simulink model "mcb_pmsm_foc_sim_RL"  (R2023a)
settings: Solver=VariableStepAuto  StartTime=0.0  StopTime=2  RelTol=1e-3
undefined symbols (not defined in the file): dataType, DiscIntNeverNeededParam, inverter, PI_params, pmsm, PU_System, Ts, Ts_agent, Ts_motor, Ts_simulink, Ts_speed
libraries: mcbcontrolslib x8, mcbpositiondecoderlib x3, simulink x2, rllib x1, mcbplantlib x1, autolibpmsmexterior x1, slpidlib x1
settings Model: Creator=The MathWorks, Inc.  LastModifiedBy=awear
settings SolverCC: AlgebraicLoopSolver=TrustRegion
settings OptimizationCC: ReuseModelBlockBuffer=off
settings DebuggingCC: ParameterPrecisionLossMsg=none  UnconnectedInputMsg=warning  UnconnectedOutputMsg=warning  UnconnectedLineMsg=warning
settings ModelReferenceCC: EnableRefExpFcnMdlSchedulingChecks=on
settings RTWCC: DLArmComputeVersion=19.05

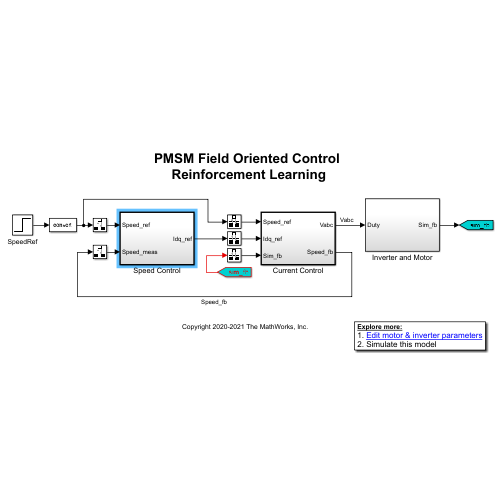
[thumbnail: Simulink's stored preview of the top-level diagram]
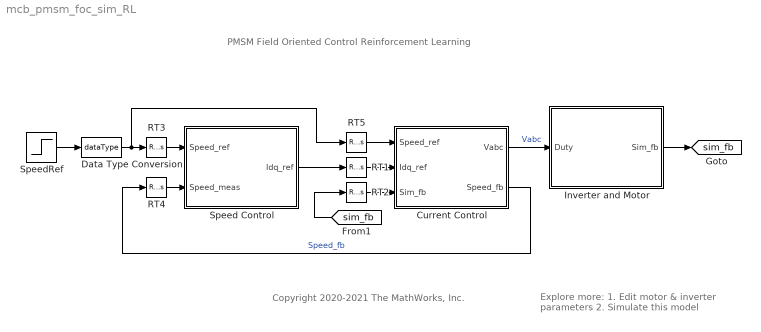
== system mcb_pmsm_foc_sim_RL ==
  note: PMSM Field Oriented Control
      | Reinforcement Learning
  note: Copyright 2020-2021 The MathWorks, Inc.
  note: Explore more:
      | 1. Edit motor & inverter parameters
      | 2. Simulate this model
  Current Control : Subsystem  TreatAsAtomicUnit=on
  Data Type Conversion : DataTypeConversion  OutDataTypeStr=dataType  SaturateOnIntegerOverflow=off  RndMeth=Floor
  Inverter and Motor : Subsystem
  RT1 : RateTransition  Deterministic=off  OutPortSampleTime=Ts
  RT2 : RateTransition  Deterministic=off  OutPortSampleTime=Ts
  RT3 : RateTransition  Deterministic=off  OutPortSampleTime=Ts_speed
  RT4 : RateTransition  Deterministic=off  OutPortSampleTime=Ts_speed
  RT5 : RateTransition  Deterministic=off  OutPortSampleTime=Ts
  Speed Control : Subsystem  TreatAsAtomicUnit=on  SystemSampleTime=Ts_speed
  SpeedRef : Step  Before=0.2  After=0.6  OutDataTypeStr=single  SampleTime=Ts_speed
  tag scope: sim_fb=global
  wires:
  Speed Control/1(Idq_ref) -> RT1/1
  RT5/1 -> Current Control/1(Speed_ref)
  SpeedRef/1 -> Data Type Conversion/1
  Current Control/2(Speed_fb) -> RT4/1  "Speed_fb"
  RT1/1 -> Current Control/2(Idq_ref)
  [sim_fb] -> RT2/1
  Data Type Conversion/1 -> RT5/1, RT3/1
  RT4/1 -> Speed Control/2(Speed_meas)
  Current Control/1(Vabc) -> Inverter and Motor/1(Duty)  "Vabc"
  RT3/1 -> Speed Control/1(Speed_ref)
  Inverter and Motor/1(Sim_fb) -> [sim_fb]
  RT2/1 -> Current Control/3(Sim_fb)

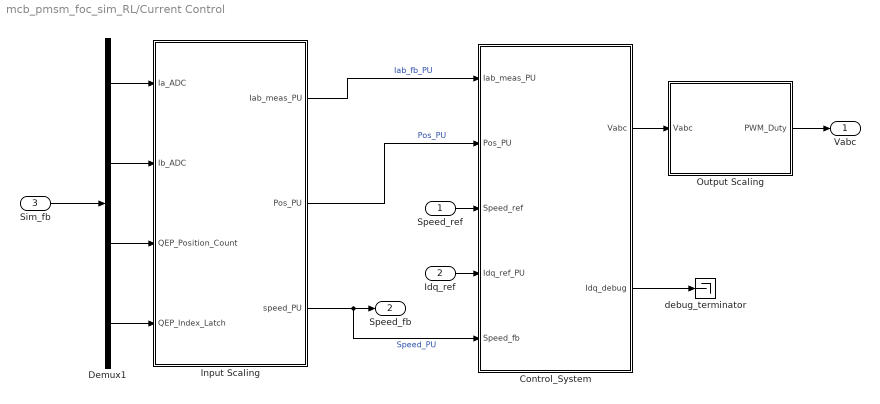
== system mcb_pmsm_foc_sim_RL/Current Control ==
  Speed_ref : Inport
  Idq_ref : Inport  Port=2
  Sim_fb : Inport  Port=3
  Control_System : Subsystem
  Demux1 : Demux
  Input Scaling : Subsystem
  Output Scaling : Subsystem
  debug_terminator : Terminator
  Vabc : Outport  InitialOutput=0  VectorParamsAs1DForOutWhenUnconnected=off
  Speed_fb : Outport  Port=2  InitialOutput=0  VectorParamsAs1DForOutWhenUnconnected=off
  wires:
  Input Scaling/2(Pos_PU) -> Control_System/2(Pos_PU)  "Pos_PU"
  Input Scaling/3(speed_PU) -> Control_System/5(Speed_fb), Speed_fb/1  "Speed_PU"
  Demux1/1 -> Input Scaling/1(Ia_ADC)
  Demux1/2 -> Input Scaling/2(Ib_ADC)
  Demux1/3 -> Input Scaling/3(QEP_Position_Count)
  Demux1/4 -> Input Scaling/4(QEP_Index_Latch)
  Control_System/2(Idq_debug) -> debug_terminator/1
  Sim_fb/1 -> Demux1/1
  Idq_ref/1 -> Control_System/4(Idq_ref_PU)
  Control_System/1(Vabc) -> Output Scaling/1(Vabc)
  Output Scaling/1(PWM_Duty) -> Vabc/1
  Input Scaling/1(Iab_meas_PU) -> Control_System/1(Iab_meas_PU)  "Iab_fb_PU"
  Speed_ref/1 -> Control_System/3(Speed_ref)

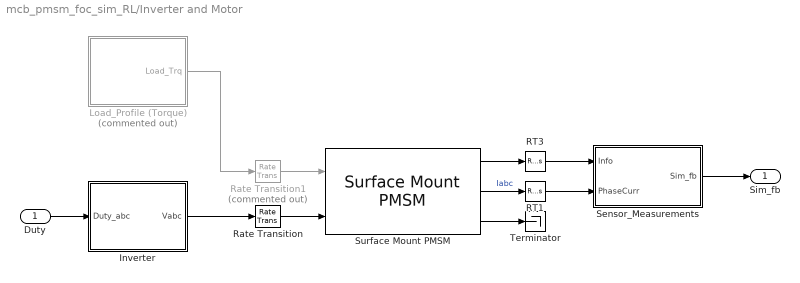
== system mcb_pmsm_foc_sim_RL/Inverter and Motor ==
  Duty : Inport
  Inverter : Subsystem
  Load_Profile (Torque) : Subsystem  Commented=on
  RT1 : RateTransition  Deterministic=off  OutPortSampleTime=Ts_simulink
  RT3 : RateTransition  Deterministic=off  OutPortSampleTime=Ts_simulink
  Rate Transition : RateTransition  Deterministic=off  OutPortSampleTime=Ts_motor
  Rate Transition1 : RateTransition  Commented=on  Deterministic=off  OutPortSampleTime=Ts_motor
  Sensor_Measurements : Subsystem
  Surface Mount PMSM : autolibpmsmexterior/Surface Mount PMSM  port_config=Torque  sim_type=Discrete  Ts=Ts_motor  P=pmsm.p  Rs=pmsm.Rs  Ldq_=pmsm.Ld  KConstText=Permanent flux linkage constant (lambda_pm):  lambda_pm=pmsm.FluxPM  Ke=159.9771  Kt=1.323  mechanical=[pmsm.J, pmsm.B, 0]  idq0=[0 0]  theta_init=0  omega_init=0  KConst=pmsm.FluxPM  lambda_pm_calc=pmsm.FluxPM  RefBlkName='autolibpmsmexterior/Surface Mount PMSM'  aMode=5  Ldq="[0.0002      0.0002]"
  Terminator : Terminator
  Sim_fb : Outport  VectorParamsAs1DForOutWhenUnconnected=off
  wires:
  Surface Mount PMSM/1 -> RT3/1
  RT1/1 -> Sensor_Measurements/2(PhaseCurr)
  RT3/1 -> Sensor_Measurements/1(Info)
  Inverter/1(Vabc) -> Rate Transition/1
  Rate Transition/1 -> Surface Mount PMSM/2
  Surface Mount PMSM/3 -> Terminator/1
  Rate Transition1/1 -> Surface Mount PMSM/1
  Sensor_Measurements/1(Sim_fb) -> Sim_fb/1
  Surface Mount PMSM/2 -> RT1/1  "Iabc"
  Load_Profile (Torque)/1(Load_Trq) -> Rate Transition1/1
  Duty/1 -> Inverter/1(Duty_abc)

== system mcb_pmsm_foc_sim_RL/Speed Control ==
  Speed_ref : Inport
  Speed_meas : Inport  Port=2
  Id_ref : Constant  Value=0  OutDataTypeStr=dataType  SampleTime=Ts_speed
  Mux1 : Mux  Inputs=2
  PI_Controller_Speed : Subsystem
  Speed Tracking : Scope  NumInputPorts=2
  Zero_Cancellation : mcbcontrolslib/IIR Filter  VariantControl=Low Pass Filter  VariantSelect=Low-pass  Filter_constant=0.01*(Ts_speed/Ts)  advancedSettings=off  Ts=50e-6  cutOff_freq=1
  Idq_ref : Outport  VectorParamsAs1DForOutWhenUnconnected=off
  wires:
  Speed_meas/1 -> Speed Tracking/2, PI_Controller_Speed/2(N_fb)  "Speed_fb"
  Id_ref/1 -> Mux1/1
  PI_Controller_Speed/1(Iq_ref) -> Mux1/2
  Mux1/1 -> Idq_ref/1
  Zero_Cancellation/1 -> PI_Controller_Speed/1(N_ref)
  Speed_ref/1 -> Speed Tracking/1, Zero_Cancellation/1  "Speed_Ref"

== system mcb_pmsm_foc_sim_RL/Current Control/Control_System ==
  Iab_meas_PU : Inport
  Pos_PU : Inport  Port=2
  Speed_ref : Inport  Port=3
  Idq_ref_PU : Inport  Port=4
  Speed_fb : Inport  Port=5
  Closed Loop Control : Subsystem
  Vabc : Outport  VectorParamsAs1DForOutWhenUnconnected=off
  Idq_debug : Outport  Port=2  VectorParamsAs1DForOutWhenUnconnected=off
  wires:
  Iab_meas_PU/1 -> Closed Loop Control/1(Iab_meas_PU)
  Pos_PU/1 -> Closed Loop Control/2(Pos_PU)
  Idq_ref_PU/1 -> Closed Loop Control/3(Idq_ref_PU)
  Closed Loop Control/1(Idq_debug) -> Idq_debug/1
  Closed Loop Control/2(Vabc in PU) -> Vabc/1
  Speed_ref/1 -> Closed Loop Control/4(Speed_ref)
  Speed_fb/1 -> Closed Loop Control/5(Speef_fb)

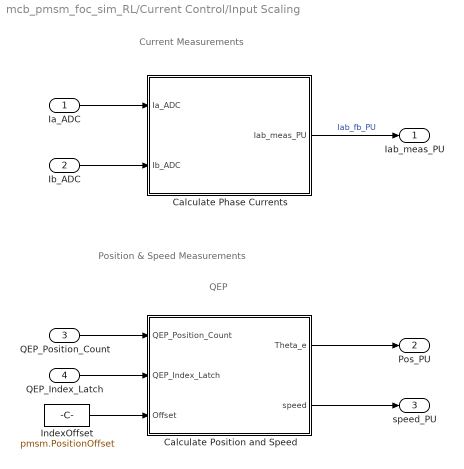
== system mcb_pmsm_foc_sim_RL/Current Control/Input Scaling ==
  note: Current Measurements
  note: Position & Speed Measurements
  note: QEP
  Ia_ADC : Inport
  Ib_ADC : Inport  Port=2
  QEP_Position_Count : Inport  Port=3
  QEP_Index_Latch : Inport  Port=4
  " Calculate Position and Speed" : Subsystem
  Calculate Phase Currents : Subsystem
  IndexOffset : Constant  Value=pmsm.PositionOffset  OutDataTypeStr=dataType  SampleTime=-1
  Iab_meas_PU : Outport
  Pos_PU : Outport  Port=2
  speed_PU : Outport  Port=3
  wires:
  " Calculate Position and Speed"/2(speed) -> speed_PU/1
  Calculate Phase Currents/1(Iab_meas_PU) -> Iab_meas_PU/1  "Iab_fb_PU"
  QEP_Position_Count/1 -> " Calculate Position and Speed"/1(QEP_Position_Count)
  " Calculate Position and Speed"/1(Theta_e) -> Pos_PU/1
  Ia_ADC/1 -> Calculate Phase Currents/1(Ia_ADC)
  Ib_ADC/1 -> Calculate Phase Currents/2(Ib_ADC)
  QEP_Index_Latch/1 -> " Calculate Position and Speed"/2(QEP_Index_Latch)
  IndexOffset/1 -> " Calculate Position and Speed"/3(Offset)

== system mcb_pmsm_foc_sim_RL/Current Control/Output Scaling ==
  Vabc : Inport
  Constant : Constant  Value=0.5  OutDataTypeStr=dataType
  Gain : Gain  Gain=0.5  OutDataTypeStr=dataType  RndMeth=Simplest
  Sum : Sum  Inputs=|++
  PWM_Duty : Outport
  wires:
  Gain/1 -> Sum/1
  Sum/1 -> PWM_Duty/1  "PWM_Duty_Cycles"
  Constant/1 -> Sum/2
  Vabc/1 -> Gain/1

== system mcb_pmsm_foc_sim_RL/Inverter and Motor/Inverter ==
  Duty_abc : Inport
  Average-Value Inverter : mcbplantlib/Average-Value Inverter
  Constant2 : Constant  Value=inverter.V_dc  OutDataTypeStr=single  SampleTime=-1
  Data Type Conversion1 : DataTypeConversion  OutDataTypeStr=single  RndMeth=Simplest  SaturateOnIntegerOverflow=off
  Rate Transition3 : RateTransition  Integrity=off  Deterministic=off  OutPortSampleTime=Ts_inverter
  Vabc : Outport  VectorParamsAs1DForOutWhenUnconnected=off
  wires:
  Constant2/1 -> Average-Value Inverter/2
  Data Type Conversion1/1 -> Rate Transition3/1
  Duty_abc/1 -> Data Type Conversion1/1
  Rate Transition3/1 -> Average-Value Inverter/1
  Average-Value Inverter/1 -> Vabc/1

== system mcb_pmsm_foc_sim_RL/Inverter and Motor/Load_Profile (Torque) ==
  Data Type Conversion : DataTypeConversion  OutDataTypeStr=single  SaturateOnIntegerOverflow=off  RndMeth=Floor
  IIR Filter : mcbcontrolslib/IIR Filter  VariantControl=Low Pass Filter  VariantSelect=Low-pass  Filter_constant=0.001  advancedSettings=off  Ts=50e-6  cutOff_freq=3.1863
  T_load : Step  Time=2  After=0  SampleTime=Ts_simulink
  Load_Trq : Outport  VectorParamsAs1DForOutWhenUnconnected=off
  wires:
  T_load/1 -> Data Type Conversion/1
  Data Type Conversion/1 -> IIR Filter/1
  IIR Filter/1 -> Load_Trq/1

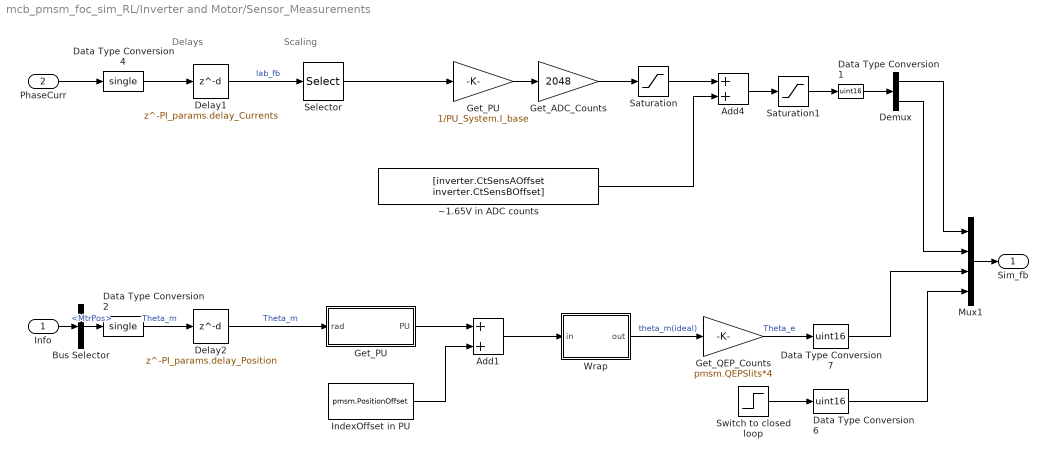
== system mcb_pmsm_foc_sim_RL/Inverter and Motor/Sensor_Measurements ==
  note: Scaling
  note: Delays
  Info : Inport
  PhaseCurr : Inport  Port=2
  Add1 : Sum  RndMeth=Simplest
  Add4 : Sum  OutDataTypeStr=uint16
  Bus Selector : BusSelector  OutputSignals=MtrPos
  Data Type Conversion1 : DataTypeConversion  OutDataTypeStr=uint16  SaturateOnIntegerOverflow=off  RndMeth=Floor
  Data Type Conversion2 : DataTypeConversion  OutDataTypeStr=single  RndMeth=Simplest  SaturateOnIntegerOverflow=off
  Data Type Conversion4 : DataTypeConversion  OutDataTypeStr=single  RndMeth=Simplest  SaturateOnIntegerOverflow=off
  Data Type Conversion6 : DataTypeConversion  OutDataTypeStr=uint16  RndMeth=Simplest  SaturateOnIntegerOverflow=off
  Data Type Conversion7 : DataTypeConversion  OutDataTypeStr=uint16  RndMeth=Simplest  SaturateOnIntegerOverflow=off
  Delay1 : Delay  DelayLength=PI_params.delay_Currents
  Delay2 : Delay  DelayLength=PI_params.delay_Position
  Demux : Demux  Outputs=2
  Get_ADC_Counts : Gain  Gain=2048  RndMeth=Simplest  OutDataTypeStr=Inherit: Same as input
  Get_PU : Gain  Gain=1/PU_System.I_base  RndMeth=Simplest
  "Get_PU " : Subsystem
  Get_QEP_Counts : Gain  Gain=pmsm.QEPSlits*4  OutDataTypeStr=uint16  RndMeth=Simplest
  IndexOffset in PU : Constant  Value=pmsm.PositionOffset  OutDataTypeStr=single  SampleTime=-1
  Mux1 : Mux
  Saturation : Saturate  UpperLimit=2048  LowerLimit=-2048
  Saturation1 : Saturate  UpperLimit=4095  LowerLimit=0
  Selector : Selector  InputPortWidth=3  IndexOptions=Index vector (dialog)  Indices=[1 2]  OutputSizes=1
  "Switch to closed loop " : Step  Time=0.1  SampleTime=Ts_motor
  Wrap : Subsystem
  ~1.65V in ADC counts : Constant  Value=[inverter.CtSensAOffset inverter.CtSensBOffset]  OutDataTypeStr=uint16  SampleTime=-1
  Sim_fb : Outport  VectorParamsAs1DForOutWhenUnconnected=off
  wires:
  Get_ADC_Counts/1 -> Saturation/1
  Saturation1/1 -> Data Type Conversion1/1
  Add4/1 -> Saturation1/1
  Data Type Conversion1/1 -> Demux/1
  ~1.65V in ADC counts/1 -> Add4/2
  Delay1/1 -> Selector/1  "Iab_fb"
  Saturation/1 -> Add4/1
  Data Type Conversion4/1 -> Delay1/1
  Selector/1 -> Get_PU/1
  PhaseCurr/1 -> Data Type Conversion4/1
  Get_PU/1 -> Get_ADC_Counts/1
  Info/1 -> Bus Selector/1
  Bus Selector/1 -> Data Type Conversion2/1  "<MtrPos>"
  Demux/1 -> Mux1/1
  Mux1/1 -> Sim_fb/1
  Demux/2 -> Mux1/2
  Data Type Conversion2/1 -> Delay2/1  "Theta_m"
  Add1/1 -> Wrap/1(in)
  Delay2/1 -> "Get_PU "/1(rad)  "Theta_m"
  Wrap/1(out) -> Get_QEP_Counts/1  "theta_m(ideal)"
  "Get_PU "/1(PU) -> Add1/1
  Get_QEP_Counts/1 -> Data Type Conversion7/1  "Theta_e"
  IndexOffset in PU/1 -> Add1/2
  Data Type Conversion7/1 -> Mux1/3
  Data Type Conversion6/1 -> Mux1/4
  "Switch to closed loop "/1 -> Data Type Conversion6/1

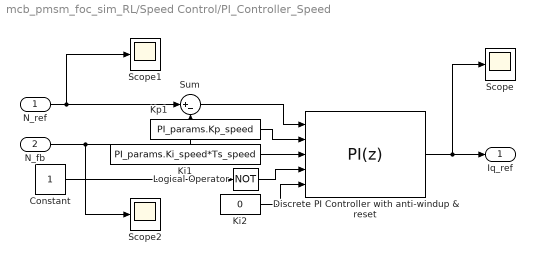
== system mcb_pmsm_foc_sim_RL/Speed Control/PI_Controller_Speed ==
  N_ref : Inport
  N_fb : Inport  Port=2
  Constant : Constant  OutDataTypeStr=boolean
  Discrete PI Controller with anti-windup & reset : slpidlib/PID Controller  Controller=PI  Form=Parallel  TimeDomain=Discrete-time  UseExternalTs=off  SampleTime=-1  IntegratorMethod=Forward Euler  FilterMethod=Forward Euler  ControllerParametersSource=external  P=1  I=1  UseKiTs=on  D=0  N=100  UseFilter=on  TunerSelectOption=Transfer Function Based (PID Tuner App)  InitialConditionSource=external  InitialConditionForIntegrator=0  InitialConditionForFilter=0  DifferentiatorICPrevScaledInput=0  ExternalReset=level  TrackingMode=off  Kt=1  LimitOutput=on  SatLimitsSource=internal  UpperSaturationLimit=1  LowerSaturationLimit=-1  LinearizeAsGain=on  AntiWindupMode=clamping  Kb=1  LimitIntegrator=off  UpperIntegratorSaturationLimit=inf  LowerIntegratorSaturationLimit=-inf  RndMeth=Simplest  POutMin=[]  POutMax=[]  IOutMin=[]  IOutMax=[]  DOutMin=[]  DOutMax=[]  NOutMin=[]  NOutMax=[]  SumOutMin=[]  SumOutMax=[]  SaturationOutDataTypeStr=Inherit: Inherit via back propagation  SaturationOutMin=[]  SaturationOutMax=[]  PParamMin=[]  PParamMax=[]  IParamMin=[]  IParamMax=[]  DParamMin=[]  DParamMax=[]  NParamMin=[]  NParamMax=[]  KbParamMin=[]  KbParamMax=[]  KtParamMin=[]  KtParamMax=[]  KbOutMin=[]  KbOutMax=[]  KtOutMin=[]  KtOutMax=[]  IntegratorOutMin=[]  IntegratorOutMax=[]  FilterOutMin=[]  FilterOutMax=[]  SumI1OutMin=[]  SumI1OutMax=[]  SumI2OutMin=[]  SumI2OutMax=[]  SumI3OutMin=[]  SumI3OutMax=[]  SumI4OutMin=[]  SumI4OutMax=[]  SumDOutMin=[]  SumDOutMax=[]  DifferentiatorOutMin=[]  DifferentiatorOutMax=[]  FilterDiffOutCoefMin=[]  FilterDiffOutCoefMax=[]  ReciprocalOutMin=[]  ReciprocalOutMax=[]  SumDenOutMin=[]  SumDenOutMax=[]  SumNumOutMin=[]  SumNumOutMax=[]  DivideOutMin=[]  DivideOutMax=[]  UdiffTsProdOutMin=[]  UdiffTsProdOutMax=[]  NTsProdOutMin=[]  NTsProdOutMax=[]  UintegralTsProdOutMin=[]  UintegralTsProdOutMax=[]  UngainTsProdOutMin=[]  UngainTsProdOutMax=[]  ClampingZeroOutDataTypeStr=Inherit: Inherit via back propagation  ClampingZeroOutMin=[]  ClampingZeroOutMax=[]  FilterDenConstantOutDataTypeStr=Inherit: Inherit via back propagation  FilterDenConstantOutMin=[]  FilterDenConstantOutMax=[]  PCopyOutDataTypeStr=Inherit: Inherit via back propagation  PCopyOutMin=[]  PCopyOutMax=[]  NCopyOutDataTypeStr=Inherit: Inherit via back propagation  NCopyOutMin=[]  NCopyOutMax=[]  IntegratorContinuousStateAttributes=''  IntegratorStateMustResolveToSignalObject=off  IntegratorRTWStateStorageClass=Auto  FilterContinuousStateAttributes=''  FilterStateMustResolveToSignalObject=off  FilterRTWStateStorageClass=Auto  ParallelPVariant=ExternalParameters  IdealPVariant=Disabled  IVariant=ExternalParameters  DVariant=Disabled  IntegratorVariant=Discrete  SatVariant=Enabled  AWVariant=DiscClampingParallel  PCopyVariant=Disabled  TRVariant=Disabled  FdbkBlocksVariant=Forward  IdealPFdbkVariant=Disabled  SatFdbkVariant=Disabled  DerivativeFilterVariant=Disabled  NVariant=Disabled  NCopyVariant=Disabled_SignalSpec  FilterICVariant=Disabled  IntegratorICVariant=ExternalICs  ExternalResetVariant=ExternalReset  TRSumVariant=Passthrough  SumFdbkVariant=Disabled  SumVariant=Sum_PI  TsampFilterVariant=InternalTs  TsampNgainVariant=Passthrough  TsampIntegralVariant=Disabled_SignalSpec  ExternalSaturationOutDataTypeStr=Inherit: Same as second input
      settings: LibrarySourceBlock=mcbcontrolslib/PI Controller
  Ki1 : Constant  Value=PI_params.Ki_speed*Ts_speed  OutDataTypeStr=dataType  SampleTime=-1
  Ki2 : Constant  Value=0  OutDataTypeStr=dataType  SampleTime=-1
  Kp1 : Constant  Value=PI_params.Kp_speed  OutDataTypeStr=dataType  SampleTime=-1
  Logical Operator : Logic  Operator=NOT  IconShape=distinctive  AllPortsSameDT=off  OutDataTypeStr=boolean
  Scope : Scope
  Scope1 : Scope
  Scope2 : Scope
  Sum : Sum  Inputs=|+-  OutDataTypeStr=Inherit: Same as first input
  Iq_ref : Outport  VectorParamsAs1DForOutWhenUnconnected=off
  wires:
  Ki1/1 -> Discrete PI Controller with anti-windup & reset/3
  Kp1/1 -> Discrete PI Controller with anti-windup & reset/2
  N_fb/1 -> Scope2/1, Sum/2
  N_ref/1 -> Sum/1, Scope1/1
  Sum/1 -> Discrete PI Controller with anti-windup & reset/1
  Logical Operator/1 -> Discrete PI Controller with anti-windup & reset/4
  Ki2/1 -> Discrete PI Controller with anti-windup & reset/5
  Constant/1 -> Logical Operator/1
  Discrete PI Controller with anti-windup & reset/1 -> Scope/1, Iq_ref/1

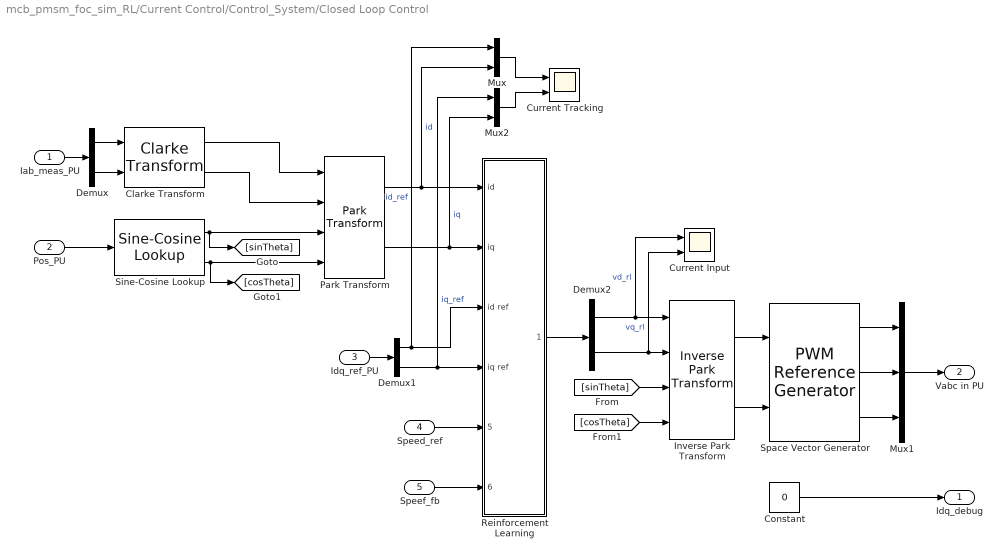
== system mcb_pmsm_foc_sim_RL/Current Control/Control_System/Closed Loop Control ==
  Iab_meas_PU : Inport
  Pos_PU : Inport  Port=2
  Idq_ref_PU : Inport  Port=3
  Speed_ref : Inport  Port=4
  Speef_fb : Inport  Port=5
  Clarke Transform : mcbcontrolslib/Clarke Transform  VariantControl=Variant2
  Constant : Constant  Value=0
  Current Input : Scope  NumInputPorts=2
  Current Tracking : Scope  NumInputPorts=2
  Demux : Demux  Outputs=2
  Demux1 : Demux  Outputs=2
  Demux2 : Demux  Outputs=2
  Inverse Park Transform : mcbcontrolslib/Inverse Park Transform  AxisAlignment=D-axis
  Mux : Mux  Inputs=2
  Mux1 : Mux  Inputs=3
  Mux2 : Mux  Inputs=2
  Park Transform : mcbcontrolslib/Park Transform  AxisAlignment=D-axis
  Reinforcement Learning : Subsystem
  Sine-Cosine Lookup : mcbcontrolslib/Sine-Cosine Lookup  AngleInput=Per-unit  N_points=1024
  Space Vector Generator : mcbcontrolslib/PWM Reference Generator  inSignal=Valphabeta  modType=SVM: space vector modulation
  Idq_debug : Outport  VectorParamsAs1DForOutWhenUnconnected=off
  Vabc in PU : Outport  Port=2  VectorParamsAs1DForOutWhenUnconnected=off
  wires:
  Sine-Cosine Lookup/1 -> [sinTheta], Park Transform/3
  Clarke Transform/2 -> Park Transform/2
  Demux/2 -> Clarke Transform/2
  Pos_PU/1 -> Sine-Cosine Lookup/1
  Demux/1 -> Clarke Transform/1
  Inverse Park Transform/2 -> Space Vector Generator/2
  Iab_meas_PU/1 -> Demux/1
  [sinTheta] -> Inverse Park Transform/3
  Inverse Park Transform/1 -> Space Vector Generator/1
  Sine-Cosine Lookup/2 -> [cosTheta], Park Transform/4
  Space Vector Generator/3 -> Mux1/3
  [cosTheta] -> Inverse Park Transform/4
  Space Vector Generator/1 -> Mux1/1
  Mux1/1 -> Vabc in PU/1
  Clarke Transform/1 -> Park Transform/1
  Space Vector Generator/2 -> Mux1/2
  Demux1/1 -> Mux/1, Reinforcement Learning/3(id ref)  "id_ref"
  Reinforcement Learning/1(action) -> Demux2/1
  Demux1/2 -> Mux2/1, Reinforcement Learning/4(iq ref)  "iq_ref"
  Idq_ref_PU/1 -> Demux1/1
  Park Transform/1 -> Reinforcement Learning/1(id), Mux/2  "id"
  Park Transform/2 -> Reinforcement Learning/2(iq), Mux2/2  "iq"
  Demux2/1 -> Current Input/1, Inverse Park Transform/1  "vd_rl"
  Demux2/2 -> Current Input/2, Inverse Park Transform/2  "vq_rl"
  Constant/1 -> Idq_debug/1
  Speed_ref/1 -> Reinforcement Learning/5(speed ref)
  Speef_fb/1 -> Reinforcement Learning/6(speed fb)
  Mux/1 -> Current Tracking/1
  Mux2/1 -> Current Tracking/2

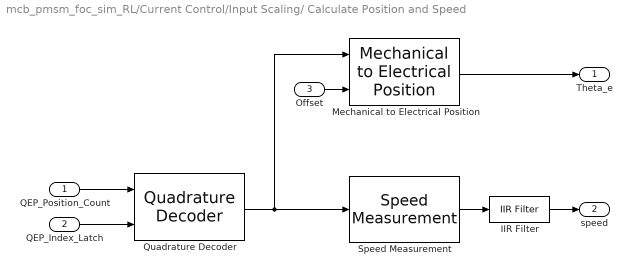
== system mcb_pmsm_foc_sim_RL/Current Control/Input Scaling/ Calculate Position and Speed ==
  QEP_Position_Count : Inport
  QEP_Index_Latch : Inport  Port=2
  Offset : Inport  Port=3
  IIR Filter : mcbcontrolslib/IIR Filter  VariantControl=Low Pass Filter  VariantSelect=Low-pass  Filter_constant=0.01  advancedSettings=off  Ts=50e-6  cutOff_freq=32.1525
  Mechanical to Electrical Position : mcbpositiondecoderlib/Mechanical to Electrical Position  NrPP=pmsm.p  selectedRange=Per unit  MechOfstInputType=Input port  mechOffsetIn=0  maxAngleIn=1  InputDataType=dataType  VariantSelect=floating-point
  Quadrature Decoder : mcbpositiondecoderlib/Quadrature Decoder  EncoderSlitsPerRevolution=pmsm.QEPSlits  EncoderCountsPerSlit=4  CounterSize=16 bits  ExternalIndexCount=on  PositionUnit=Per unit  PositionDataType=dataType
  Speed Measurement : mcbpositiondecoderlib/Speed Measurement  PositionUnit=Per unit  PositionScalingDatatype=uint32  SpeedCalculationMode=Time interval for speed calculation  SampleTimeAsync=Ts  MaximumApplicationSpeed=6000  SpeedResolution=5e-6  DelayLength=20  MaximumMeasurableSpeed=7499  MeasurableSpeedResolution=3.4925e-06  SpeedUnit=Per unit based on dialog  PerUnitSpeed=PU_System.N_base  SpeedDataType=dataType
  Theta_e : Outport  VectorParamsAs1DForOutWhenUnconnected=off
  speed : Outport  Port=2  VectorParamsAs1DForOutWhenUnconnected=off
  wires:
  Speed Measurement/1 -> IIR Filter/1
  Mechanical to Electrical Position/1 -> Theta_e/1
  QEP_Position_Count/1 -> Quadrature Decoder/1
  Quadrature Decoder/1 -> Speed Measurement/1, Mechanical to Electrical Position/1
  Offset/1 -> Mechanical to Electrical Position/2
  IIR Filter/1 -> speed/1
  QEP_Index_Latch/1 -> Quadrature Decoder/2

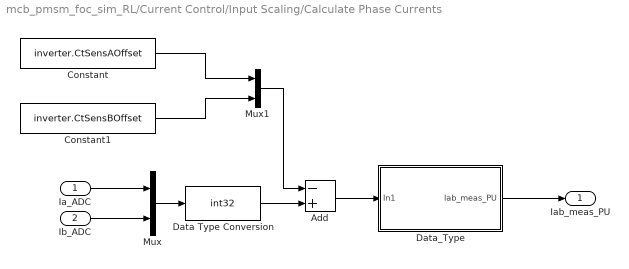
== system mcb_pmsm_foc_sim_RL/Current Control/Input Scaling/Calculate Phase Currents ==
  Ia_ADC : Inport
  Ib_ADC : Inport  Port=2
  Add : Sum  Inputs=-+
  Constant : Constant  Value=inverter.CtSensAOffset  OutDataTypeStr=uint16
  Constant1 : Constant  Value=inverter.CtSensBOffset  OutDataTypeStr=uint16
  Data Type Conversion : DataTypeConversion  OutDataTypeStr=int32  ConvertRealWorld=Stored Integer (SI)  RndMeth=Simplest  SaturateOnIntegerOverflow=off
  Data_Type : Subsystem  Variant=on
  Mux : Mux  Inputs=2
  Mux1 : Mux  Inputs=2
  Iab_meas_PU : Outport  VectorParamsAs1DForOutWhenUnconnected=off
  wires:
  Data Type Conversion/1 -> Add/2
  Add/1 -> Data_Type/1(In1)
  Data_Type/1(Iab_meas_PU) -> Iab_meas_PU/1
  Ia_ADC/1 -> Mux/1
  Ib_ADC/1 -> Mux/2
  Mux/1 -> Data Type Conversion/1
  Constant/1 -> Mux1/1
  Constant1/1 -> Mux1/2
  Mux1/1 -> Add/1

== system mcb_pmsm_foc_sim_RL/Inverter and Motor/Sensor_Measurements/Get_PU  ==
  rad : Inport
  Constant2 : Constant  Value=2*pi  OutDataTypeStr=single  SampleTime=-1
  Get_PU : Gain  Gain=1/(2*pi)  RndMeth=Simplest  OutDataTypeStr=Inherit: Same as input
  Mod : Math  Operator=mod
  PU : Outport  VectorParamsAs1DForOutWhenUnconnected=off
  wires:
  rad/1 -> Mod/1
  Constant2/1 -> Mod/2
  Mod/1 -> Get_PU/1
  Get_PU/1 -> PU/1

== system mcb_pmsm_foc_sim_RL/Inverter and Motor/Sensor_Measurements/Wrap ==
  in : Inport
  Constant2 : Constant  OutDataTypeStr=single  SampleTime=-1
  Mod : Math  Operator=mod
  out : Outport  VectorParamsAs1DForOutWhenUnconnected=off
  wires:
  in/1 -> Mod/1
  Constant2/1 -> Mod/2
  Mod/1 -> out/1

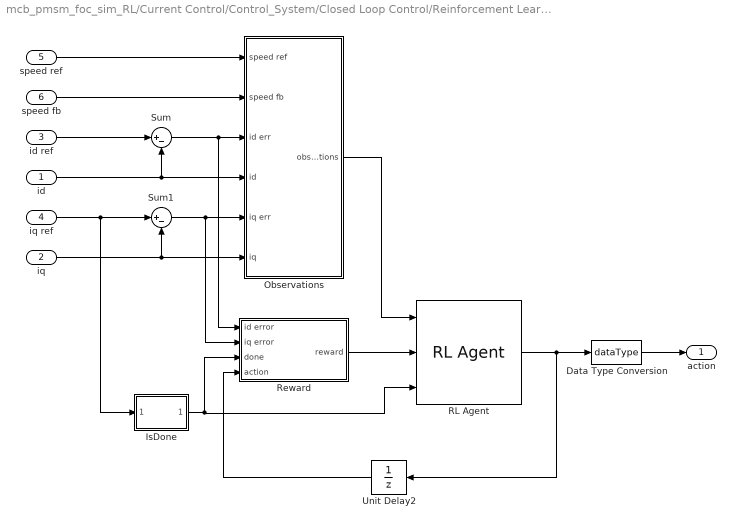
== system mcb_pmsm_foc_sim_RL/Current Control/Control_System/Closed Loop Control/Reinforcement Learning ==
  id : Inport
  iq : Inport  Port=2
  id ref : Inport  Port=3
  iq ref : Inport  Port=4
  speed ref : Inport  Port=5
  speed fb : Inport  Port=6
  Data Type Conversion : DataTypeConversion  OutDataTypeStr=dataType  SaturateOnIntegerOverflow=off  RndMeth=Floor
  IsDone : Subsystem
  Observations : Subsystem
  RL Agent : rllib/RL Agent  Agent=agent  ExternalActionAsInput=off  ProvideLastAction=off  ProvideCumRwd=off  TreatAsDirectFeedthrough=on  UseStrictObservationDataTypes=off
  Reward : Subsystem
  Sum : Sum  Inputs=|+-  OutDataTypeStr=Inherit: Inherit via back propagation
  Sum1 : Sum  Inputs=|+-  OutDataTypeStr=Inherit: Inherit via back propagation
  Unit Delay2 : UnitDelay  SampleTime=-1  HasFrameUpgradeWarning=on
  action : Outport
  wires:
  Observations/1(observations) -> RL Agent/1
  Reward/1(reward) -> RL Agent/2
  RL Agent/1 -> Data Type Conversion/1, Unit Delay2/1
  Data Type Conversion/1 -> action/1
  speed ref/1 -> Observations/1(speed ref)
  speed fb/1 -> Observations/2(speed fb)
  Unit Delay2/1 -> Reward/4(action)
  IsDone/1(stop) -> RL Agent/3, Reward/3(done)
  id ref/1 -> Sum/1
  id/1 -> Sum/2, Observations/4(id)
  Sum/1 -> Reward/1(id error), Observations/3(id err)
  Sum1/1 -> Reward/2(iq error), Observations/5(iq err)
  iq ref/1 -> IsDone/1(Iq_ref), Sum1/1
  iq/1 -> Sum1/2, Observations/6(iq)

== system mcb_pmsm_foc_sim_RL/Current Control/Input Scaling/Calculate Phase Currents/Data_Type ==
  In1 : Inport
  Data_Type_Fixed_Point : Subsystem  VariantControl=~isequal(dataType,'single')
  Data_Type_Float : Subsystem  VariantControl=isequal(dataType,'single')
  Iab_meas_PU : Outport

== system mcb_pmsm_foc_sim_RL/Current Control/Control_System/Closed Loop Control/Reinforcement Learning/IsDone ==
  Iq_ref : Inport
  Compare To Constant2 : simulink/Logic and Bit Operations/Compare To Constant  relop=>=  const=0.3  OutDataTypeStr=boolean
  Compare To Constant3 : simulink/Logic and Bit Operations/Compare To Constant  relop=>=  const=1  OutDataTypeStr=boolean
  Digital Clock : DigitalClock  SampleTime=Ts_agent
  OR1 : Logic  IconShape=distinctive  AllPortsSameDT=off  OutDataTypeStr=boolean
  Product : Product
  TrainFlag : Constant  Value=0  OutDataTypeStr=double
  stop : Outport
  wires:
  Compare To Constant2/1 -> OR1/2
  Iq_ref/1 -> Compare To Constant3/1
  Compare To Constant3/1 -> OR1/1
  OR1/1 -> Product/1
  Digital Clock/1 -> Compare To Constant2/1
  Product/1 -> stop/1
  TrainFlag/1 -> Product/2

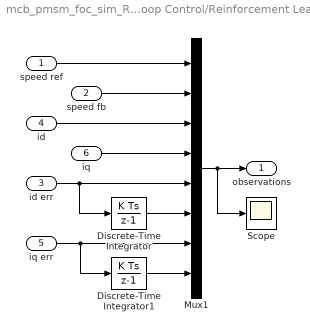
== system mcb_pmsm_foc_sim_RL/Current Control/Control_System/Closed Loop Control/Reinforcement Learning/Observations ==
  speed ref : Inport
  speed fb : Inport  Port=2
  id err : Inport  Port=3
  id : Inport  Port=4
  iq err : Inport  Port=5
  iq : Inport  Port=6
  Discrete-Time Integrator : DiscreteIntegrator  SampleTime=-1  ICPrevOutput=DiscIntNeverNeededParam  ICPrevScaledInput=DiscIntNeverNeededParam
  Discrete-Time Integrator1 : DiscreteIntegrator  SampleTime=-1  ICPrevOutput=DiscIntNeverNeededParam  ICPrevScaledInput=DiscIntNeverNeededParam
  Mux1 : Mux  Inputs=8
  Scope : Scope
  observations : Outport  VectorParamsAs1DForOutWhenUnconnected=off
  wires:
  speed ref/1 -> Mux1/1
  speed fb/1 -> Mux1/2
  id/1 -> Mux1/3
  iq/1 -> Mux1/4
  Mux1/1 -> Scope/1, observations/1
  Discrete-Time Integrator1/1 -> Mux1/8
  iq err/1 -> Mux1/7, Discrete-Time Integrator1/1
  Discrete-Time Integrator/1 -> Mux1/6
  id err/1 -> Mux1/5, Discrete-Time Integrator/1

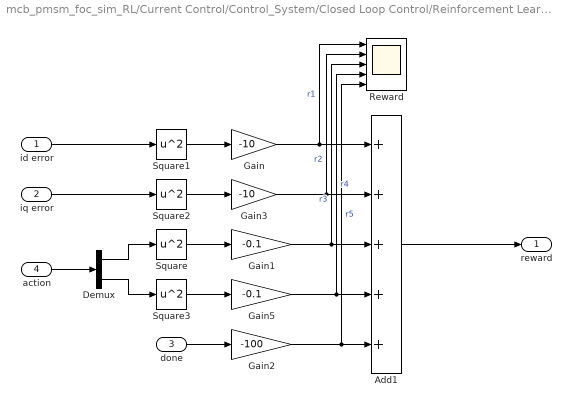
== system mcb_pmsm_foc_sim_RL/Current Control/Control_System/Closed Loop Control/Reinforcement Learning/Reward ==
  id error : Inport
  iq error : Inport  Port=2
  done : Inport  Port=3
  action : Inport  Port=4
  Add1 : Sum  Inputs=+++++
  Demux : Demux  Outputs=2
  Gain : Gain  Gain=-10
  Gain1 : Gain  Gain=-0.1
  Gain2 : Gain  Gain=-100
  Gain3 : Gain  Gain=-10
  Gain5 : Gain  Gain=-0.1
  Reward : Scope  NumInputPorts=5
  Square{,1..3} (4 alike) : Math  Operator=square
  reward : Outport  VectorParamsAs1DForOutWhenUnconnected=off
  wires:
  Square1/1 -> Gain/1
  Square2/1 -> Gain3/1
  Demux/1 -> Square/1
  Square/1 -> Gain1/1
  Gain1/1 -> Reward/3, Add1/3  "r3"
  Demux/2 -> Square3/1
  Square3/1 -> Gain5/1
  action/1 -> Demux/1
  Add1/1 -> reward/1
  Gain5/1 -> Reward/4, Add1/4  "r4"
  Gain/1 -> Reward/1, Add1/1  "r1"
  Gain3/1 -> Reward/2, Add1/2  "r2"
  id error/1 -> Square1/1
  iq error/1 -> Square2/1
  Gain2/1 -> Add1/5, Reward/5  "r5"
  done/1 -> Gain2/1

== system mcb_pmsm_foc_sim_RL/Current Control/Input Scaling/Calculate Phase Currents/Data_Type/Data_Type_Fixed_Point ==
  In1 : Inport
  Data Type Conversion : DataTypeConversion  OutDataTypeStr=fixdt(1,32,17)  ConvertRealWorld=Stored Integer (SI)  RndMeth=Simplest  SaturateOnIntegerOverflow=off
  Data Type Conversion1 : DataTypeConversion  OutDataTypeStr=dataType  RndMeth=Simplest  SaturateOnIntegerOverflow=off
  Q17 per unit conversion : ArithShift  BitShiftNumber=-6
  Iab_meas_PU : Outport
  wires:
  In1/1 -> Q17 per unit conversion/1
  Data Type Conversion1/1 -> Iab_meas_PU/1
  Data Type Conversion/1 -> Data Type Conversion1/1
  Q17 per unit conversion/1 -> Data Type Conversion/1

== system mcb_pmsm_foc_sim_RL/Current Control/Input Scaling/Calculate Phase Currents/Data_Type/Data_Type_Float ==
  In1 : Inport
  Current Sense Gain : Gain  Gain=PU_System.I_base/1.65  RndMeth=Simplest  OutDataTypeStr=Inherit: Same as input
  Get_ADC_Volt : Gain  Gain=1.65/2048  OutDataTypeStr=dataType  RndMeth=Simplest
  PU_Conversion : Gain  Gain=1/PU_System.I_base  RndMeth=Simplest  OutDataTypeStr=Inherit: Same as input
  Iab_meas_PU : Outport
  wires:
  Current Sense Gain/1 -> PU_Conversion/1
  In1/1 -> Get_ADC_Volt/1
  Get_ADC_Volt/1 -> Current Sense Gain/1
  PU_Conversion/1 -> Iab_meas_PU/1
